simulink model "final_project_full_working"  (R2024b)
settings: Solver=ode1  StartTime=0.0  StopTime=5  RelTol=1e-4  AbsTol=1e-3
undefined symbols (not defined in the file): DiscIntNeverNeededParam, Ion, Lithium
libraries: spsSeriesRLCBranchLib x25, slpidlib x12, spsThreePhaseVIMeasurementLib x11, spsPower3phInstantaneousLib x9, spsIGBTDiodeLib x7, spsThreePhaseParallelRLCLoadLib x7, spsCurrentMeasurementLib x4, spsabctodq0Lib x3, spsVoltageMeasurementLib x3, spsGroundLib x3, spsVariableResistorLib x3, spsControlledVoltageSourceLib x3
(part 1 of 2)
settings Model: Creator=ALVEE  LastModifiedBy=ALVEE
settings SolverCC: SolverResetMethod=Robust

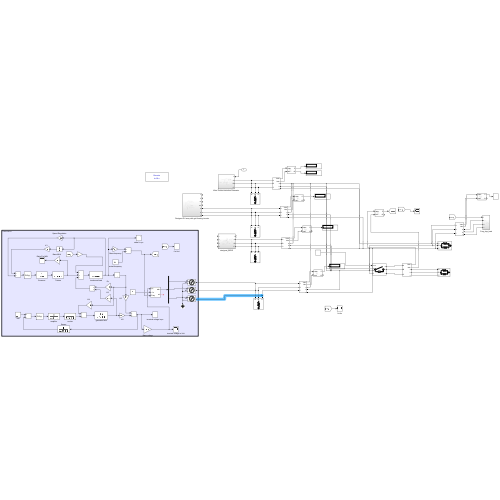
[thumbnail: Simulink's stored preview of the top-level diagram]
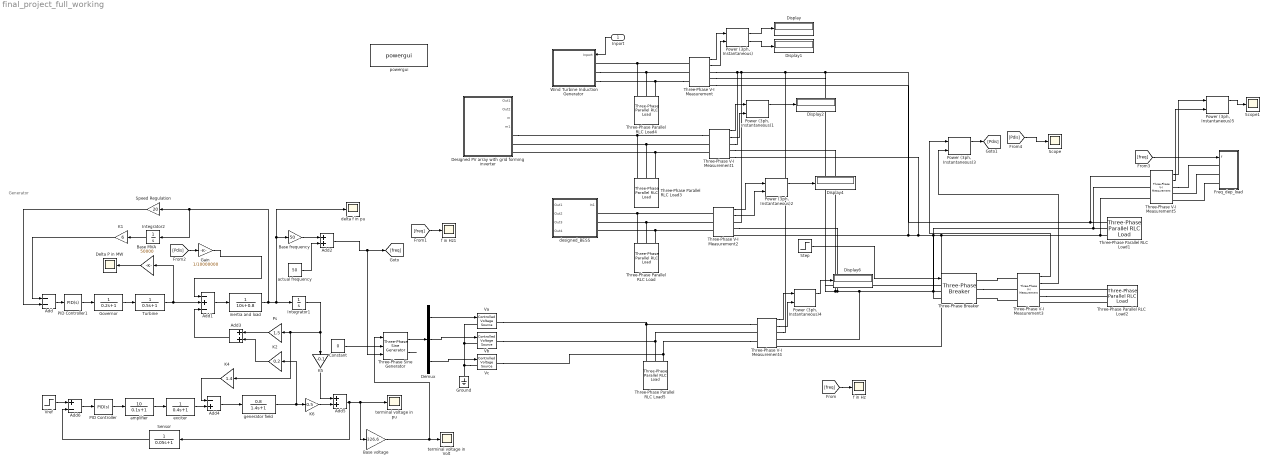
== system final_project_full_working ==
  note: Generator
  Inport : Inport
  Add : Sum  Inputs=--
  Add1 : Sum  Inputs=-+-
  Add2 : Sum
  Add3 : Sum
  Add4 : Sum  Inputs=-+
  Add5 : Sum
  Add6 : Sum  Inputs=+-
  Base MVA : Gain  Gain=50000
  Base frequency : Gain  Gain=50
  Base voltage : Gain  Gain=326.6
  Constant : Constant  Value=0
  Delta P in MW : Scope
  Demux : Demux  Outputs=3
  Designed PV array with grid forming inverter : Subsystem
  Display{,1..2,4,6} (5 alike) : Display
  Freq_dep_load : Subsystem
  Gain : Gain  Gain=1/10000000
  Governor : TransferFcn  Denominator=[0.2 1]
  Ground : spsGroundLib/Ground  LConnTagsString=a
  Integrator1 : Integrator
  Integrator2 : Integrator
  K1 : Gain  Gain=6
  K2 : Gain  Gain=0.2
  K4 : Gain  Gain=1.4
  K5 : Gain  Gain=-0.1
  K6 : Gain  Gain=0.5
  PID Controller : slpidlib/PID Controller  Controller=PID  Form=Parallel  TimeDomain=Continuous-time  UseExternalTs=off  SampleTime=-1  IntegratorMethod=Forward Euler  FilterMethod=Forward Euler  ControllerParametersSource=internal  P=1  I=0.25  UseKiTs=off  D=0.3  UseExternalDerivativeSource=off  N=100  UseFilter=on  TunerSelectOption=Transfer Function Based (PID Tuner App)  InitialConditionSource=internal  InitialConditionForIntegrator=0  InitialConditionForFilter=0  DifferentiatorICPrevScaledInput=0  ExternalReset=none  TrackingMode=off  Kt=1  LimitOutput=off  SatLimitsSource=internal  UpperSaturationLimit=inf  LowerSaturationLimit=-inf  LinearizeAsGain=on  AntiWindupMode=none  Kb=1  LimitIntegrator=off  UpperIntegratorSaturationLimit=inf  LowerIntegratorSaturationLimit=-inf  POutMin=[]  POutMax=[]  IOutMin=[]  IOutMax=[]  DOutMin=[]  DOutMax=[]  NOutMin=[]  NOutMax=[]  SumOutMin=[]  SumOutMax=[]  SaturationOutMin=[]  SaturationOutMax=[]  PParamMin=[]  PParamMax=[]  IParamMin=[]  IParamMax=[]  DParamMin=[]  DParamMax=[]  NParamMin=[]  NParamMax=[]  KbParamMin=[]  KbParamMax=[]  KtParamMin=[]  KtParamMax=[]  KbOutMin=[]  KbOutMax=[]  KtOutMin=[]  KtOutMax=[]  IntegratorOutMin=[]  IntegratorOutMax=[]  FilterOutMin=[]  FilterOutMax=[]  SumI1OutMin=[]  SumI1OutMax=[]  SumI2OutMin=[]  SumI2OutMax=[]  SumI3OutMin=[]  SumI3OutMax=[]  SumI4OutMin=[]  SumI4OutMax=[]  SumDOutMin=[]  SumDOutMax=[]  DifferentiatorOutMin=[]  DifferentiatorOutMax=[]  FilterDiffOutCoefMin=[]  FilterDiffOutCoefMax=[]  ReciprocalOutMin=[]  ReciprocalOutMax=[]  SumDenOutMin=[]  SumDenOutMax=[]  SumNumOutMin=[]  SumNumOutMax=[]  DivideOutMin=[]  DivideOutMax=[]  UdiffTsProdOutMin=[]  UdiffTsProdOutMax=[]  NTsProdOutMin=[]  NTsProdOutMax=[]  UintegralTsProdOutMin=[]  UintegralTsProdOutMax=[]  UngainTsProdOutMin=[]  UngainTsProdOutMax=[]  ClampingZeroOutDataTypeStr=Inherit: Inherit via back propagation  ClampingZeroOutMin=[]  ClampingZeroOutMax=[]  FilterDenConstantOutDataTypeStr=Inherit: Inherit via back propagation  FilterDenConstantOutMin=[]  FilterDenConstantOutMax=[]  PCopyOutDataTypeStr=Inherit: Inherit via back propagation  PCopyOutMin=[]  PCopyOutMax=[]  NCopyOutDataTypeStr=Inherit: Inherit via back propagation  NCopyOutMin=[]  NCopyOutMax=[]  IntegratorContinuousStateAttributes=''  IntegratorStateMustResolveToSignalObject=off  IntegratorRTWStateStorageClass=Auto  FilterContinuousStateAttributes=''  FilterStateMustResolveToSignalObject=off  FilterRTWStateStorageClass=Auto  ParallelPVariant=InternalParameters  IdealPVariant=Disabled  IVariant=InternalParameters  DVariant=InternalParameters  IntegratorVariant=Continuous  SatVariant=Disabled  AWVariant=Passthrough  PCopyVariant=Disabled  TRVariant=Disabled  FdbkBlocksVariant=Forward  IdealPFdbkVariant=Disabled  SatFdbkVariant=Disabled  DerivativeFilterVariant=ContFilter  NVariant=InternalParameters  NCopyVariant=Disabled  FilterICVariant=InternalICsFilter  IntegratorICVariant=InternalICs  ExternalResetVariant=Disabled  TRSumVariant=Passthrough  SumFdbkVariant=Disabled  SumVariant=Sum_PID  TsampFilterVariant=InternalTs  TsampNgainVariant=Passthrough  TsampIntegralVariant=Disabled_SignalSpec  ExternalSaturationOutDataTypeStr=Inherit: Same as second input  DerivativeSourceVariant=ErrorSignal  PreIntVariant=InternalPreInt
  PID Controller1 : slpidlib/PID Controller  Controller=PID  Form=Parallel  TimeDomain=Continuous-time  UseExternalTs=off  SampleTime=-1  IntegratorMethod=Forward Euler  FilterMethod=Forward Euler  ControllerParametersSource=internal  P=24.0972  I=15.6479  UseKiTs=off  D=10  UseExternalDerivativeSource=off  N=100  UseFilter=on  TunerSelectOption=Transfer Function Based (PID Tuner App)  InitialConditionSource=internal  InitialConditionForIntegrator=0  InitialConditionForFilter=0  DifferentiatorICPrevScaledInput=0  ExternalReset=none  TrackingMode=off  Kt=1  LimitOutput=off  SatLimitsSource=internal  UpperSaturationLimit=inf  LowerSaturationLimit=-inf  LinearizeAsGain=on  AntiWindupMode=none  Kb=1  LimitIntegrator=off  UpperIntegratorSaturationLimit=inf  LowerIntegratorSaturationLimit=-inf  POutMin=[]  POutMax=[]  IOutMin=[]  IOutMax=[]  DOutMin=[]  DOutMax=[]  NOutMin=[]  NOutMax=[]  SumOutMin=[]  SumOutMax=[]  SaturationOutMin=[]  SaturationOutMax=[]  PParamMin=[]  PParamMax=[]  IParamMin=[]  IParamMax=[]  DParamMin=[]  DParamMax=[]  NParamMin=[]  NParamMax=[]  KbParamMin=[]  KbParamMax=[]  KtParamMin=[]  KtParamMax=[]  KbOutMin=[]  KbOutMax=[]  KtOutMin=[]  KtOutMax=[]  IntegratorOutMin=[]  IntegratorOutMax=[]  FilterOutMin=[]  FilterOutMax=[]  SumI1OutMin=[]  SumI1OutMax=[]  SumI2OutMin=[]  SumI2OutMax=[]  SumI3OutMin=[]  SumI3OutMax=[]  SumI4OutMin=[]  SumI4OutMax=[]  SumDOutMin=[]  SumDOutMax=[]  DifferentiatorOutMin=[]  DifferentiatorOutMax=[]  FilterDiffOutCoefMin=[]  FilterDiffOutCoefMax=[]  ReciprocalOutMin=[]  ReciprocalOutMax=[]  SumDenOutMin=[]  SumDenOutMax=[]  SumNumOutMin=[]  SumNumOutMax=[]  DivideOutMin=[]  DivideOutMax=[]  UdiffTsProdOutMin=[]  UdiffTsProdOutMax=[]  NTsProdOutMin=[]  NTsProdOutMax=[]  UintegralTsProdOutMin=[]  UintegralTsProdOutMax=[]  UngainTsProdOutMin=[]  UngainTsProdOutMax=[]  ClampingZeroOutDataTypeStr=Inherit: Inherit via back propagation  ClampingZeroOutMin=[]  ClampingZeroOutMax=[]  FilterDenConstantOutDataTypeStr=Inherit: Inherit via back propagation  FilterDenConstantOutMin=[]  FilterDenConstantOutMax=[]  PCopyOutDataTypeStr=Inherit: Inherit via back propagation  PCopyOutMin=[]  PCopyOutMax=[]  NCopyOutDataTypeStr=Inherit: Inherit via back propagation  NCopyOutMin=[]  NCopyOutMax=[]  IntegratorContinuousStateAttributes=''  IntegratorStateMustResolveToSignalObject=off  IntegratorRTWStateStorageClass=Auto  FilterContinuousStateAttributes=''  FilterStateMustResolveToSignalObject=off  FilterRTWStateStorageClass=Auto  ParallelPVariant=InternalParameters  IdealPVariant=Disabled  IVariant=InternalParameters  DVariant=InternalParameters  IntegratorVariant=Continuous  SatVariant=Disabled  AWVariant=Passthrough  PCopyVariant=Disabled  TRVariant=Disabled  FdbkBlocksVariant=Forward  IdealPFdbkVariant=Disabled  SatFdbkVariant=Disabled  DerivativeFilterVariant=ContFilter  NVariant=InternalParameters  NCopyVariant=Disabled  FilterICVariant=InternalICsFilter  IntegratorICVariant=InternalICs  ExternalResetVariant=Disabled  TRSumVariant=Passthrough  SumFdbkVariant=Disabled  SumVariant=Sum_PID  TsampFilterVariant=InternalTs  TsampNgainVariant=Passthrough  TsampIntegralVariant=Disabled_SignalSpec  ExternalSaturationOutDataTypeStr=Inherit: Same as second input  DerivativeSourceVariant=ErrorSignal  PreIntVariant=InternalPreInt
  Power (3ph, Instantaneous){,1..5} (6 alike) : spsPower3phInstantaneousLib/Power (3ph, Instantaneous)
  Ps : Gain  Gain=1.5
  Scope : Scope
  Scope1 : Scope
  Sensor : TransferFcn  Denominator=[0.05 1]
  Speed Regulation : Gain  Gain=20
  Step : Step  Time=2.5  SampleTime=0
  Three-Phase Parallel RLC Load{,3..5} (4 alike) : spsThreePhaseParallelRLCLoadLib/Three-Phase Parallel RLC Load  LConnTagsString=A|B|C  Configuration=Y (grounded)  NominalVoltage=400  Vabc=[1e3 1e3 1e3]  Vabcp=[1e3 1e3 1e3]  NominalFrequency=50  UnbalancedPower=off  ActivePower=100  InductivePower=0  CapacitivePower=0  Pabc=[10e3 9e3 11e3]  QLabc=[100 90 110]  QCabc=[100 90 110]  Pabcp=[10e3 9e3 11e3]  QLabcp=[100 90 110]  QCabcp=[100 90 110]  Measurements=None  LoadType=constant Z
  Three-Phase Parallel RLC Load1 : spsThreePhaseParallelRLCLoadLib/Three-Phase Parallel RLC Load  LConnTagsString=A|B|C  Configuration=Y (grounded)  NominalVoltage=400  Vabc=[1e3 1e3 1e3]  Vabcp=[1e3 1e3 1e3]  NominalFrequency=50  UnbalancedPower=off  ActivePower=10e6  InductivePower=100  CapacitivePower=0  Pabc=[10e3 9e3 11e3]  QLabc=[100 90 110]  QCabc=[100 90 110]  Pabcp=[10e3 9e3 11e3]  QLabcp=[100 90 110]  QCabcp=[100 90 110]  Measurements=None  LoadType=constant PQ
  Three-Phase Parallel RLC Load2 : spsThreePhaseParallelRLCLoadLib/Three-Phase Parallel RLC Load  LConnTagsString=A|B|C  Configuration=Y (grounded)  NominalVoltage=400  Vabc=[1e3 1e3 1e3]  Vabcp=[1e3 1e3 1e3]  NominalFrequency=50  UnbalancedPower=off  ActivePower=2e6  InductivePower=100  CapacitivePower=0  Pabc=[10e3 9e3 11e3]  QLabc=[100 90 110]  QCabc=[100 90 110]  Pabcp=[10e3 9e3 11e3]  QLabcp=[100 90 110]  QCabcp=[100 90 110]  Measurements=None  LoadType=constant PQ
  Three-Phase Sine Generator : spsThreePhaseSineGeneratorLib/Three-Phase Sine Generator  Ts=0.0002
      settings: LibrarySourceBlock=|
      | sps_lib/Sources/Signal Generator Sources/Three-Phase
      | Sine Generator
  Three-Phase V-I Measurement{,1..5} (6 alike) : spsThreePhaseVIMeasurementLib/Three-Phase V-I Measurement  VoltageMeasurement=phase-to-ground  SetLabelV=off  LabelV=Vabc  Vpu=off  VpuLL=off  CurrentMeasurement=yes  SetLabelI=off  LabelI=Iabc  Ipu=off  Pbase=100e6  Vbase=500e3  OutputType=Complex  PhasorSimulation=off  PSBequivalent=0
  Three-Phase Breaker : spsThreePhaseBreakerLib/Three-Phase Breaker  InitialState=open  SwitchA=on  SwitchB=on  SwitchC=on  SwitchTimes="[1/60  5/60]"  External=on  BreakerResistance=0.01  SnubberResistance=1e6  SnubberCapacitance=inf  Measurements=None
  Turbine : TransferFcn  Denominator=[0.5 1]
  Va : spsControlledVoltageSourceLib/Controlled Voltage Source  Initialize=on  Source_Type=AC  Amplitude=0  Phase=0  Frequency=0  Measurements=None
  Vb : spsControlledVoltageSourceLib/Controlled Voltage Source  Initialize=on  Source_Type=AC  Amplitude=0  Phase=0  Frequency=0  Measurements=None
  Vc : spsControlledVoltageSourceLib/Controlled Voltage Source  Initialize=on  Source_Type=AC  Amplitude=0  Phase=0  Frequency=0  Measurements=None
  Vref : Step  Time=100  Before=1  SampleTime=0
  Wind Turbine Induction Generator : Subsystem
  actual frequency : Constant  Value=50
  amplifier : TransferFcn  Numerator=[10]  Denominator=[0.1 1]
  delta f in pu : Scope
  designed_BESS : Subsystem
  exciter : TransferFcn  Denominator=[0.4 1]
  f in Hz : Scope
  f in Hz1 : Scope
  generator field : TransferFcn  Numerator=[0.8]  Denominator=[1.4 1]
  inertia and load : TransferFcn  Denominator=[10 0.8]
  powergui : spspowerguiLib/powergui  Priority=1  SimulationMode=Discrete  SampleTime=1e-5  frequency=60  Iterations=50  frequencyindice=0  Pbase=100e6  ErrMax=1e-4  UnitsV=kV  UnitsW=MW  buscounter=0  FunctionMessages=off  echomessages=off  EnableUseOfTLC=off  CurrentSourceSwitches=off  DisableSnubberDevices=off  DisableRonSwitches=off  DisableVfSwitches=off  DisplayEquations=off  AutomaticDiscreteSolvers=off  SolverType=Tustin/Backward Euler (TBE)  Interpol=off  ExternalGateDelay=off  methode=off  Ts=100  x0status=blocks  SPID=on  SwTol=0  HookPort=off  NonlinearTolerance=1e-4  nMaxIteration=100  ContinueOnMaxIteration=off  RestoreLinks=warning  ResistiveCurrentMeasurement=off  Frange=[0:2:500]  Ylog=off  Xlog=on  ShowGrid=off  save=off  variable=ZData  structure=0  ZoomFFT=off  StartTime=0.0  cycles=1  DisplayStyle=1  fundamental=60  FreqAxis=off  MaxFrequency=1000  frequencyindicesteady=1  RmsSteady=1  display=off
  terminal voltage in Volt : Scope
  terminal voltage in pu : Scope
  wires:
  Three-Phase Sine Generator/2 -> ?
  Add3/1 -> Add1/3
  actual frequency/1 -> Add2/2
  inertia and load/1 -> Base frequency/1, delta f in pu/1, Integrator1/1, Speed Regulation/1, Integrator2/1
  K6/1 -> Add5/2
  Three-Phase V-I Measurement3/1 -> "Power (3ph, Instantaneous)3"/1
  PID Controller/1 -> amplifier/1
  Demux/3 -> Vc/1
  K2/1 -> Add3/2
  Base MVA/1 -> Delta P in MW/1
  Governor/1 -> Turbine/1
  Three-Phase V-I Measurement2/2 -> "Power (3ph, Instantaneous)2"/2
  Demux/2 -> Vb/1
  Sensor/1 -> Add6/2
  "Power (3ph, Instantaneous)"/2 -> Display1/1
  [freq] -> f in Hz1/1
  [Pdis] -> Gain/1
  Add4/1 -> generator field/1
  Integrator2/1 -> K1/1
  Turbine/1 -> Add1/2, Base MVA/1
  "Power (3ph, Instantaneous)"/1 -> Display/1
  Three-Phase V-I Measurement1/2 -> "Power (3ph, Instantaneous)1"/2
  Speed Regulation/1 -> Add/2
  Inport/1 -> Wind Turbine Induction Generator/1(Inport)
  Three-Phase Sine Generator/1 -> Demux/1
  "Power (3ph, Instantaneous)4"/1 -> Display6/1
  [Pdis] -> Scope/1
  "Power (3ph, Instantaneous)2"/1 -> Display4/1
  K4/1 -> Add4/1
  Integrator1/1 -> K5/1, K4/1, Ps/1
  "Power (3ph, Instantaneous)1"/1 -> Display2/1
  generator field/1 -> K2/1, K6/1
  "Power (3ph, Instantaneous)3"/1 -> [Pdis]
  Three-Phase V-I Measurement1/1 -> "Power (3ph, Instantaneous)1"/1
  Add2/1 -> Three-Phase Sine Generator/3, [freq]
  Constant/1 -> Three-Phase Sine Generator/2
  Three-Phase V-I Measurement/1 -> "Power (3ph, Instantaneous)"/1
  Three-Phase V-I Measurement2/1 -> "Power (3ph, Instantaneous)2"/1
  exciter/1 -> Add4/2
  Three-Phase V-I Measurement4/1 -> "Power (3ph, Instantaneous)4"/1
  Base frequency/1 -> Add2/1
  Ps/1 -> Add3/1
  [freq] -> Freq_dep_load/1(f)
  Three-Phase V-I Measurement4/2 -> "Power (3ph, Instantaneous)4"/2
  Base voltage/1 -> Three-Phase Sine Generator/1, terminal voltage in Volt/1
  Gain/1 -> Add1/1
  Vref/1 -> Add6/1
  [freq] -> f in Hz/1
  Add1/1 -> inertia and load/1
  Demux/1 -> Va/1
  K1/1 -> Add/1
  Add6/1 -> PID Controller/1
  Three-Phase V-I Measurement3/2 -> "Power (3ph, Instantaneous)3"/2
  Add5/1 -> Base voltage/1, terminal voltage in pu/1, Sensor/1
  Three-Phase V-I Measurement5/1 -> "Power (3ph, Instantaneous)5"/1
  "Power (3ph, Instantaneous)5"/1 -> Scope1/1
  Three-Phase V-I Measurement/2 -> "Power (3ph, Instantaneous)"/2
  Three-Phase V-I Measurement5/2 -> "Power (3ph, Instantaneous)5"/2
  Step/1 -> Three-Phase Breaker/1
  amplifier/1 -> exciter/1
  K5/1 -> Add5/1
  Add/1 -> PID Controller1/1
  PID Controller1/1 -> Governor/1
  connections:
  Three-Phase Parallel RLC Load3/LConn3 -- Three-Phase V-I Measurement1/LConn3 -- Designed PV array with grid forming inverter/RConn3
  Three-Phase V-I Measurement1/RConn3 -- Three-Phase Breaker/LConn3 -- Three-Phase V-I Measurement5/LConn3 -- Three-Phase Parallel RLC Load1/LConn3 -- Three-Phase V-I Measurement4/RConn3 -- Three-Phase V-I Measurement/RConn3 -- Three-Phase V-I Measurement2/RConn3
  Three-Phase V-I Measurement/LConn3 -- Wind Turbine Induction Generator/LConn3 -- Three-Phase Parallel RLC Load4/LConn3
  Three-Phase V-I Measurement2/RConn1 -- Three-Phase V-I Measurement5/LConn1 -- Three-Phase Parallel RLC Load1/LConn1 -- Three-Phase Breaker/LConn1 -- Three-Phase V-I Measurement4/RConn1 -- Three-Phase V-I Measurement/RConn1 -- Three-Phase V-I Measurement1/RConn1
  Three-Phase V-I Measurement4/LConn3 -- Three-Phase Parallel RLC Load5/LConn3 -- Vc/RConn1
  Vc/LConn1 -- Va/LConn1 -- Vb/LConn1 -- Ground/LConn1
  Three-Phase V-I Measurement2/RConn2 -- Three-Phase V-I Measurement5/LConn2 -- Three-Phase Parallel RLC Load1/LConn2 -- Three-Phase Breaker/LConn2 -- Three-Phase V-I Measurement4/RConn2 -- Three-Phase V-I Measurement/RConn2 -- Three-Phase V-I Measurement1/RConn2
  Three-Phase V-I Measurement4/LConn1 -- Three-Phase Parallel RLC Load5/LConn1 -- Va/RConn1
  designed_BESS/LConn1 -- Three-Phase V-I Measurement2/LConn1 -- Three-Phase Parallel RLC Load/LConn1
  Three-Phase Parallel RLC Load/LConn2 -- Three-Phase V-I Measurement2/LConn2 -- designed_BESS/LConn2
  Three-Phase V-I Measurement1/LConn1 -- Designed PV array with grid forming inverter/RConn1 -- Three-Phase Parallel RLC Load3/LConn1
  Three-Phase Parallel RLC Load/LConn3 -- Three-Phase V-I Measurement2/LConn3 -- designed_BESS/LConn3
  Three-Phase Parallel RLC Load4/LConn2 -- Wind Turbine Induction Generator/LConn2 -- Three-Phase V-I Measurement/LConn2
  Wind Turbine Induction Generator/LConn1 -- Three-Phase V-I Measurement/LConn1 -- Three-Phase Parallel RLC Load4/LConn1
  Three-Phase Parallel RLC Load3/LConn2 -- Three-Phase V-I Measurement1/LConn2 -- Designed PV array with grid forming inverter/RConn2
  Vb/RConn1 -- Three-Phase V-I Measurement4/LConn2 -- Three-Phase Parallel RLC Load5/LConn2
  Three-Phase Breaker/RConn2 -- Three-Phase V-I Measurement3/LConn2
  Freq_dep_load/LConn3 -- Three-Phase V-I Measurement5/RConn3
  Three-Phase Parallel RLC Load2/LConn3 -- Three-Phase V-I Measurement3/RConn3
  Three-Phase V-I Measurement3/LConn1 -- Three-Phase Breaker/RConn1
  Three-Phase V-I Measurement5/RConn1 -- Freq_dep_load/LConn1
  Three-Phase Parallel RLC Load2/LConn1 -- Three-Phase V-I Measurement3/RConn1
  Three-Phase V-I Measurement3/LConn3 -- Three-Phase Breaker/RConn3
  Three-Phase V-I Measurement3/RConn2 -- Three-Phase Parallel RLC Load2/LConn2
  Freq_dep_load/LConn2 -- Three-Phase V-I Measurement5/RConn2

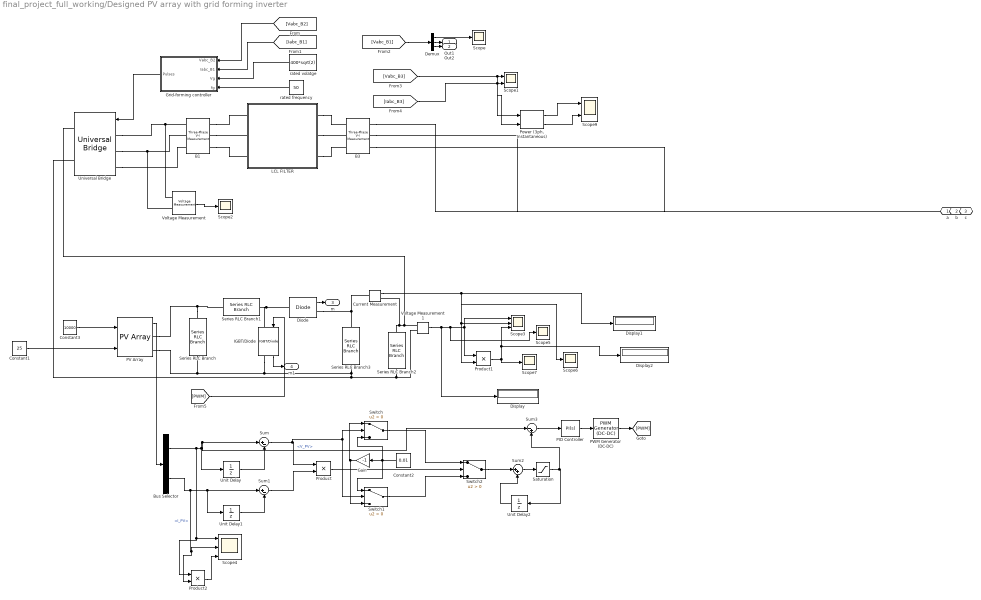
== system final_project_full_working/Designed PV array with grid forming inverter ==
  B1 : spsThreePhaseVIMeasurementLib/Three-Phase V-I Measurement  VoltageMeasurement=phase-to-ground  SetLabelV=on  LabelV=Vabc_B1  Vpu=off  VpuLL=off  CurrentMeasurement=yes  SetLabelI=on  LabelI=Iabc_B1  Ipu=off  Pbase=100e6  Vbase=500e3  OutputType=Complex  PhasorSimulation=off  PSBequivalent=0
  B3 : spsThreePhaseVIMeasurementLib/Three-Phase V-I Measurement  VoltageMeasurement=phase-to-ground  SetLabelV=on  LabelV=Vabc_B3  Vpu=off  VpuLL=off  CurrentMeasurement=yes  SetLabelI=on  LabelI=Iabc_B3  Ipu=off  Pbase=100e6  Vbase=500e3  OutputType=Complex  PhasorSimulation=off  PSBequivalent=0
  Bus Selector : BusSelector  OutputSignals=V_PV,I_PV
  Constant1 : Constant  Value=25
  Constant2 : Constant  Value=0.01
  Constant3 : Constant  Value=10000
  Current Measurement : spsCurrentMeasurementLib/Current Measurement  PhasorSimulation=off  OutputType=Complex  PSBequivalent=0
  Demux : Demux  Outputs=3
  Diode : spsDiodeLib/Diode  Ron=0.01  Lon=0  Vf=0.8  IC=0  UseSnubber=0  Rs=500  Cs=250e-9  Measurements=on
  Display : Display
  Display1 : Display
  Display2 : Display
  Gain : Gain  Gain=-1
  Grid-forming controller : Subsystem
  IGBT/Diode : spsIGBTDiodeLib/IGBT//Diode  Ron=1e-3  Rs=1e5  Cs=inf  Measurements=on
  LCL FILTER : Subsystem
  PID Controller : slpidlib/PID Controller  Controller=PI  Form=Parallel  TimeDomain=Continuous-time  UseExternalTs=off  SampleTime=-1  IntegratorMethod=Forward Euler  FilterMethod=Forward Euler  ControllerParametersSource=internal  P=1  I=1  UseKiTs=off  D=0  UseExternalDerivativeSource=off  N=100  UseFilter=on  TunerSelectOption=Transfer Function Based (PID Tuner App)  InitialConditionSource=internal  InitialConditionForIntegrator=0  InitialConditionForFilter=0  DifferentiatorICPrevScaledInput=0  ExternalReset=none  TrackingMode=off  Kt=1  LimitOutput=off  SatLimitsSource=internal  UpperSaturationLimit=inf  LowerSaturationLimit=-inf  LinearizeAsGain=on  AntiWindupMode=none  Kb=1  LimitIntegrator=off  UpperIntegratorSaturationLimit=inf  LowerIntegratorSaturationLimit=-inf  POutMin=[]  POutMax=[]  IOutMin=[]  IOutMax=[]  DOutMin=[]  DOutMax=[]  NOutMin=[]  NOutMax=[]  SumOutMin=[]  SumOutMax=[]  SaturationOutMin=[]  SaturationOutMax=[]  PParamMin=[]  PParamMax=[]  IParamMin=[]  IParamMax=[]  DParamMin=[]  DParamMax=[]  NParamMin=[]  NParamMax=[]  KbParamMin=[]  KbParamMax=[]  KtParamMin=[]  KtParamMax=[]  KbOutMin=[]  KbOutMax=[]  KtOutMin=[]  KtOutMax=[]  IntegratorOutMin=[]  IntegratorOutMax=[]  FilterOutMin=[]  FilterOutMax=[]  SumI1OutMin=[]  SumI1OutMax=[]  SumI2OutMin=[]  SumI2OutMax=[]  SumI3OutMin=[]  SumI3OutMax=[]  SumI4OutMin=[]  SumI4OutMax=[]  SumDOutMin=[]  SumDOutMax=[]  DifferentiatorOutMin=[]  DifferentiatorOutMax=[]  FilterDiffOutCoefMin=[]  FilterDiffOutCoefMax=[]  ReciprocalOutMin=[]  ReciprocalOutMax=[]  SumDenOutMin=[]  SumDenOutMax=[]  SumNumOutMin=[]  SumNumOutMax=[]  DivideOutMin=[]  DivideOutMax=[]  UdiffTsProdOutMin=[]  UdiffTsProdOutMax=[]  NTsProdOutMin=[]  NTsProdOutMax=[]  UintegralTsProdOutMin=[]  UintegralTsProdOutMax=[]  UngainTsProdOutMin=[]  UngainTsProdOutMax=[]  ClampingZeroOutDataTypeStr=Inherit: Inherit via back propagation  ClampingZeroOutMin=[]  ClampingZeroOutMax=[]  FilterDenConstantOutDataTypeStr=Inherit: Inherit via back propagation  FilterDenConstantOutMin=[]  FilterDenConstantOutMax=[]  PCopyOutDataTypeStr=Inherit: Inherit via back propagation  PCopyOutMin=[]  PCopyOutMax=[]  NCopyOutDataTypeStr=Inherit: Inherit via back propagation  NCopyOutMin=[]  NCopyOutMax=[]  IntegratorContinuousStateAttributes=''  IntegratorStateMustResolveToSignalObject=off  IntegratorRTWStateStorageClass=Auto  FilterContinuousStateAttributes=''  FilterStateMustResolveToSignalObject=off  FilterRTWStateStorageClass=Auto  ParallelPVariant=InternalParameters  IdealPVariant=Disabled  IVariant=InternalParameters  DVariant=Disabled  IntegratorVariant=Continuous  SatVariant=Disabled  AWVariant=Passthrough  PCopyVariant=Disabled  TRVariant=Disabled  FdbkBlocksVariant=Forward  IdealPFdbkVariant=Disabled  SatFdbkVariant=Disabled  DerivativeFilterVariant=Disabled  NVariant=Disabled  NCopyVariant=Disabled_SignalSpec  FilterICVariant=Disabled  IntegratorICVariant=InternalICs  ExternalResetVariant=Disabled  TRSumVariant=Passthrough  SumFdbkVariant=Disabled  SumVariant=Sum_PI  TsampFilterVariant=InternalTs  TsampNgainVariant=Passthrough  TsampIntegralVariant=Disabled_SignalSpec  ExternalSaturationOutDataTypeStr=Inherit: Same as second input  DerivativeSourceVariant=Disabled  PreIntVariant=InternalPreInt
  PV Array : spsPVArrayLib/PV Array  Npar=1000  Nser=100  PlotType=array @ 25 deg.C & specified irradiances  S_vec="[ 1000  500  100 ]"  Temp_C_vec="[ 45 25  ]"  ModuleName=SunPower SPR-445J-WHT-D  PlotWhenSelected=off  Pm=444.86  Ncell=128  Voc=90.5  Isc=6.21  Vm=76.7  Im=5.8  beta_Voc_pc=-0.291  alpha_Isc_pc=0.013301  beta_Voc=-0.26336  alpha_Isc=0.000826  IL=6.2167  I0=1.3548e-11  nI=1.026  Rsh=508.2885  Rs=0.54863  RobustModel=off  RobustCellTemperature=313.3991  BAL=on  Tc=1e-6  Tfilter=5e-5
  PWM Generator (DC-DC) : spsPWMGeneratorDCDCLib/PWM Generator (DC-DC)  Fsw=10000  Ts=0
  "Power (3ph, Instantaneous)" : spsPower3phInstantaneousLib/Power (3ph, Instantaneous)
  Product : Product
  Product1 : Product
  Product2 : Product
  Saturation : Saturate  UpperLimit=400  LowerLimit=350
  Scope{,2,5..7} (5 alike) : Scope
  Scope1 : Scope  NumInputPorts=2
  Scope3 : Scope  NumInputPorts=3
  Scope4 : Scope  NumInputPorts=3
  Scope9 : Scope  NumInputPorts=2
  Series RLC Branch : spsSeriesRLCBranchLib/Series RLC Branch  LConnTagsString=__new0  RConnTagsString=__new0  BranchType=C  Resistance=1  Inductance=1e-3  SetiL0=off  InitialCurrent=0  Capacitance=1.5625e-3  Setx0=off  InitialVoltage=0  Measurements=None
  Series RLC Branch1 : spsSeriesRLCBranchLib/Series RLC Branch  LConnTagsString=__new0  RConnTagsString=__new0  BranchType=L  Resistance=1  Inductance=0.1024  SetiL0=off  InitialCurrent=0  Capacitance=1e-6  Setx0=off  InitialVoltage=0  Measurements=None
  Series RLC Branch2 : spsSeriesRLCBranchLib/Series RLC Branch  LConnTagsString=__new0  RConnTagsString=__new0  BranchType=R  Resistance=0.15994  Inductance=1e-3  SetiL0=off  InitialCurrent=0  Capacitance=1e-6  Setx0=off  InitialVoltage=0  Measurements=None
  Series RLC Branch3 : spsSeriesRLCBranchLib/Series RLC Branch  LConnTagsString=__new0  RConnTagsString=__new0  BranchType=C  Resistance=1  Inductance=1e-3  SetiL0=off  InitialCurrent=0  Capacitance=0.015625  Setx0=off  InitialVoltage=0  Measurements=None
  Sum : Sum  Inputs=|+-
  Sum1 : Sum  Inputs=|+-
  Sum2 : Sum  Inputs=|++
  Sum3 : Sum  Inputs=|-+
  Switch : Switch  Criteria=u2 > Threshold  SaturateOnIntegerOverflow=off  InputSameDT=off
  Switch1 : Switch  Criteria=u2 > Threshold  SaturateOnIntegerOverflow=off  InputSameDT=off
  Switch2 : Switch  Criteria=u2 > Threshold  SaturateOnIntegerOverflow=off  InputSameDT=off
  Unit Delay : UnitDelay  SampleTime=-1  HasFrameUpgradeWarning=on
  Unit Delay1 : UnitDelay  SampleTime=-1  HasFrameUpgradeWarning=on
  Unit Delay2 : UnitDelay  SampleTime=-1  HasFrameUpgradeWarning=on
  Universal Bridge : spsUniversalBridgeLib/Universal Bridge  Arms=3  SnubberResistance=1e5  SnubberCapacitance=inf  Device=IGBT / Diodes  Ron=1e-3  Lon=0  ForwardVoltages="[  0  0  ]"  ForwardVoltage=0  GTOparameters=[ 10e-6 , 20e-6 ]  IGBTparameters=[ 1e-6 , 2e-6 ]  Measurements=None  Measurements_2=None  converterType=Rectifier
  Voltage Measurement : spsVoltageMeasurementLib/Voltage Measurement  PhasorSimulation=off  OutputType=Complex  PSBequivalent=0
  Voltage Measurement1 : spsVoltageMeasurementLib/Voltage Measurement  PhasorSimulation=off  OutputType=Complex  PSBequivalent=0
  rated frequency : Constant  Value=50  SampleTime=10e-6
  rated volatge : Constant  Value=400*sqrt(2)  SampleTime=10e-6
  a : PMIOPort  Side=Right
  b : PMIOPort  Port=2  Side=Right
  c : PMIOPort  Port=3  Side=Right
  Out1 : Outport
  Out2 : Outport  Port=2
  m : Outport  Port=3
  m1 : Outport  Port=4
  wires:
  Bus Selector/1 -> Product2/1, Scope4/1, Unit Delay/1, Sum3/1, Sum/1  "<V_PV>"
  Current Measurement/1 -> Display1/1, Product1/2, Scope3/2, Scope6/1
  Product/1 -> Switch2/2
  Demux/1 -> Scope/1
  Product1/1 -> Display2/1, Scope3/3, Scope7/1
  Constant2/1 -> Switch1/1, Switch/3, Gain/1
  Sum/1 -> Switch1/2, Switch/2, Product/1
  [Vabc_B2] -> Grid-forming controller/1(Vabc_B2)
  Sum3/1 -> PID Controller/1
  rated volatge/1 -> Grid-forming controller/3(Vg)
  Voltage Measurement1/1 -> Display/1, Scope5/1, Scope3/1, Product1/1
  [Iabc_B3] -> "Power (3ph, Instantaneous)"/2, Scope1/2
  "Power (3ph, Instantaneous)"/2 -> Scope9/2
  Bus Selector/2 -> Product2/2, Scope4/2, Unit Delay1/1, Sum1/1  "<I_PV>"
  Unit Delay/1 -> Sum/2
  PID Controller/1 -> PWM Generator (DC-DC)/1
  [Iabc_B1] -> Grid-forming controller/2(Iabc_B1)
  Gain/1 -> Switch1/3, Switch/1
  [PWM] -> IGBT/Diode/1
  Unit Delay2/1 -> Sum2/2
  Grid-forming controller/1(Pulses) -> Universal Bridge/1
  PV Array/1 -> Bus Selector/1
  Switch2/1 -> Sum2/1
  Saturation/1 -> Sum3/2, Unit Delay2/1
  Constant3/1 -> PV Array/1
  [Vabc_B3] -> "Power (3ph, Instantaneous)"/1, Scope1/1
  PWM Generator (DC-DC)/1 -> [PWM]
  "Power (3ph, Instantaneous)"/1 -> Scope9/1
  Diode/1 -> m/1
  Unit Delay1/1 -> Sum1/2
  Constant1/1 -> PV Array/2
  [Vabc_B1] -> Demux/1
  Demux/2 -> Out1/1
  Switch/1 -> Switch2/1
  Product2/1 -> Scope4/3
  Demux/3 -> Out2/1
  rated frequency/1 -> Grid-forming controller/4(fg)
  Switch1/1 -> Switch2/3
  IGBT/Diode/1 -> m1/1
  Voltage Measurement/1 -> Scope2/1
  Sum1/1 -> Product/2
  Sum2/1 -> Saturation/1
  connections:
  Series RLC Branch2/RConn1 -- Universal Bridge/RConn2 -- Series RLC Branch3/RConn1 -- IGBT/Diode/RConn1 -- PV Array/RConn2 -- Series RLC Branch/RConn1 -- Voltage Measurement1/LConn2
  Universal Bridge/LConn2 -- Voltage Measurement/LConn2 -- B1/LConn2
  Diode/RConn1 -- Current Measurement/LConn1 -- Series RLC Branch3/LConn1
  Series RLC Branch/LConn1 -- PV Array/RConn1 -- Series RLC Branch1/LConn1
  Universal Bridge/LConn3 -- B1/LConn3
  B1/RConn3 -- LCL FILTER/LConn3
  B3/RConn2 -- b/RConn1
  Diode/LConn1 -- IGBT/Diode/LConn1 -- Series RLC Branch1/RConn1
  B3/RConn1 -- a/RConn1
  Universal Bridge/LConn1 -- Voltage Measurement/LConn1 -- B1/LConn1
  LCL FILTER/RConn1 -- B3/LConn1
  LCL FILTER/RConn2 -- B3/LConn2
  B1/RConn1 -- LCL FILTER/LConn1
  B1/RConn2 -- LCL FILTER/LConn2
  LCL FILTER/RConn3 -- B3/LConn3
  Current Measurement/RConn1 -- Universal Bridge/RConn1 -- Voltage Measurement1/LConn1 -- Series RLC Branch2/LConn1
  B3/RConn3 -- c/RConn1

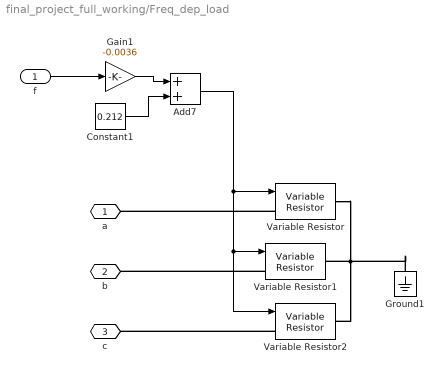
== system final_project_full_working/Freq_dep_load ==
  f : Inport
  Add7 : Sum
  Constant1 : Constant  Value=0.212
  Gain1 : Gain  Gain=-0.0036
  Ground1 : spsGroundLib/Ground  LConnTagsString=a
  Variable Resistor : spsVariableResistorLib/Variable Resistor  Rabsmin=1e-3
  Variable Resistor1 : spsVariableResistorLib/Variable Resistor  Rabsmin=1e-3
  Variable Resistor2 : spsVariableResistorLib/Variable Resistor  Rabsmin=1e-3
  a : PMIOPort  Side=Left
  " b" : PMIOPort  Port=2  Side=Left
  " c" : PMIOPort  Port=3  Side=Left
  wires:
  f/1 -> Gain1/1
  Constant1/1 -> Add7/2
  Add7/1 -> Variable Resistor2/1, Variable Resistor1/1, Variable Resistor/1
  Gain1/1 -> Add7/1
  connections:
  Variable Resistor/RConn1 -- Variable Resistor2/RConn1 -- Ground1/LConn1 -- Variable Resistor1/RConn1
  Variable Resistor2/LConn1 -- " c"/RConn1
  Variable Resistor/LConn1 -- a/RConn1
  Variable Resistor1/LConn1 -- " b"/RConn1

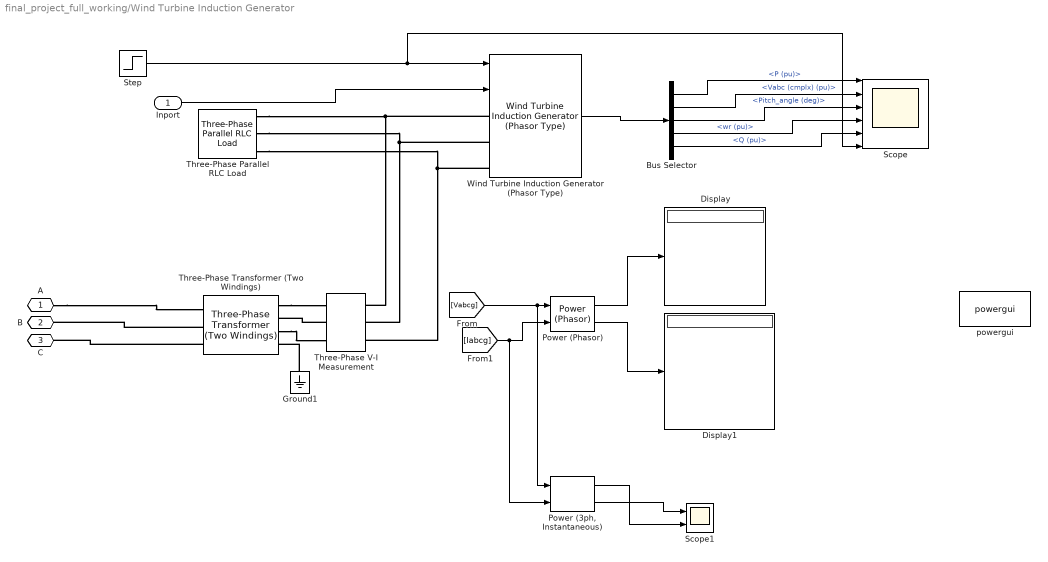
== system final_project_full_working/Wind Turbine Induction Generator ==
  Inport : Inport
  Bus Selector : BusSelector  OutputSignals=P (pu),Vabc (cmplx) (pu),Pitch_angle (deg),wr (pu),Q (pu)
  Display : Display
  Display1 : Display
  Ground1 : spsGroundLib/Ground  LConnTagsString=a
  "Power (3ph, Instantaneous)" : spsPower3phInstantaneousLib/Power (3ph, Instantaneous)
  Power (Phasor) : spsPowerPhasorLib/Power (Phasor)
  Scope : Scope  NumInputPorts=6
  Scope1 : Scope  NumInputPorts=2
  Step : Step  Time=2.5  Before=12  After=12.5  SampleTime=0
  Three-Phase Parallel RLC Load : spsThreePhaseParallelRLCLoadLib/Three-Phase Parallel RLC Load  LConnTagsString=A|B|C  Configuration=Y (grounded)  NominalVoltage=400  Vabc=[1e3 1e3 1e3]  Vabcp=[1e3 1e3 1e3]  NominalFrequency=50  UnbalancedPower=off  ActivePower=0  InductivePower=0  CapacitivePower=5000  Pabc=[10e3 9e3 11e3]  QLabc=[100 90 110]  QCabc=[100 90 110]  Pabcp=[10e3 9e3 11e3]  QLabcp=[100 90 110]  QCabcp=[100 90 110]  Measurements=None  LoadType=constant Z
  Three-Phase Transformer (Two Windings) : spsThreePhaseTransformerTwoWindingsLib/Three-Phase Transformer (Two Windings)  Winding1Connection=Yg  Winding2Connection=Yn  CoreType=Three single-phase transformers  SetSaturation=off  Hysteresis=off  DataFile='hysteresis'  SetInitialFlux=off  Measurements=None  UNITS=pu  NominalPower=[ 15e3 , 50 ]  Winding1=[ 400 , 0.002 , 0.08 ]  Winding2=[ 400 , 0.002 , 0.08 ]  Rm=500  Lm=inf  L0=0.5  Saturation=[ 0,0 ; 0.0024,1.2 ; 1.0,1.52 ]  InitialFluxes=[ 0.8 , -0.8 , 0.7 ]  BreakLoop=off  DiscreteSolver=Trapezoidal iterative  DataType=off  TransfoNumber=1
  Three-Phase V-I Measurement : spsThreePhaseVIMeasurementLib/Three-Phase V-I Measurement  VoltageMeasurement=phase-to-ground  SetLabelV=on  LabelV=Vabcg  Vpu=off  VpuLL=off  CurrentMeasurement=yes  SetLabelI=on  LabelI=Iabcg  Ipu=off  Pbase=100e6  Vbase=500e3  OutputType=Complex  PhasorSimulation=off  PSBequivalent=0
  Wind Turbine Induction Generator (Phasor Type) : spsWindTurbineInductionGeneratorPhasorTypeLib/Wind Turbine Induction Generator (Phasor Type)  ExternalTm=off  nom=[10e3, 400, 50]  sta=[ 0.004843, 0.1248]  rot=[ 0.004377, 0.1791]  Lm=6.77  mec=[5.04, 0.01, 3]  init="[ -0.01,0,   0,0,0,   0,0,0 ]"  pitch_angle=0  Pmec=1e4  wind_base=12  speed_nom=1  P_wind_base=1  K_pitch_gain=[5 25]  pitch_max=45  pitch_rate=2
  powergui : spspowerguiLib/powergui  Priority=1  SimulationMode=Discrete  SampleTime=1e-5  frequency=50  Iterations=50  frequencyindice=50  Pbase=100e6  ErrMax=1e-4  UnitsV=kV  UnitsW=MW  buscounter=0  FunctionMessages=off  echomessages=off  EnableUseOfTLC=off  CurrentSourceSwitches=off  DisableSnubberDevices=off  DisableRonSwitches=off  DisableVfSwitches=off  DisplayEquations=off  AutomaticDiscreteSolvers=off  SolverType=Tustin/Backward Euler (TBE)  Interpol=off  ExternalGateDelay=off  methode=off  Ts=100  x0status=blocks  SPID=on  SwTol=0  HookPort=off  NonlinearTolerance=1e-4  nMaxIteration=100  ContinueOnMaxIteration=off  RestoreLinks=warning  ResistiveCurrentMeasurement=off  Frange=[0:2:500]  Ylog=off  Xlog=on  ShowGrid=off  save=off  variable=ZData  structure=0  ZoomFFT=off  StartTime=0.0  cycles=1  DisplayStyle=1  fundamental=60  FreqAxis=off  MaxFrequency=1000  frequencyindicesteady=1  RmsSteady=1  display=off
  A : PMIOPort  Side=Left
  B : PMIOPort  Port=2  Side=Left
  C : PMIOPort  Port=3  Side=Left
  wires:
  Bus Selector/5 -> Scope/5  "<Q (pu)>"
  Bus Selector/1 -> Scope/1  "<P (pu)>"
  Wind Turbine Induction Generator (Phasor Type)/1 -> Bus Selector/1
  Power (Phasor)/2 -> Display1/1
  [Iabcg] -> "Power (3ph, Instantaneous)"/2, Power (Phasor)/2
  [Vabcg] -> "Power (3ph, Instantaneous)"/1, Power (Phasor)/1
  Bus Selector/3 -> Scope/3  "<Pitch_angle (deg)>"
  Step/1 -> Scope/6, Wind Turbine Induction Generator (Phasor Type)/1
  Power (Phasor)/1 -> Display/1
  Inport/1 -> Wind Turbine Induction Generator (Phasor Type)/2
  Bus Selector/2 -> Scope/2  "<Vabc (cmplx) (pu)>"
  Bus Selector/4 -> Scope/4  "<wr (pu)>"
  "Power (3ph, Instantaneous)"/1 -> Scope1/2
  "Power (3ph, Instantaneous)"/2 -> Scope1/1
  connections:
  Three-Phase Transformer (Two Windings)/RConn1 -- Three-Phase V-I Measurement/LConn1
  Ground1/LConn1 -- Three-Phase Transformer (Two Windings)/RConn4
  Wind Turbine Induction Generator (Phasor Type)/LConn3 -- Three-Phase Parallel RLC Load/LConn3 -- Three-Phase V-I Measurement/RConn3
  A/RConn1 -- Three-Phase Transformer (Two Windings)/LConn1
  Wind Turbine Induction Generator (Phasor Type)/LConn2 -- Three-Phase Parallel RLC Load/LConn2 -- Three-Phase V-I Measurement/RConn2
  Three-Phase Transformer (Two Windings)/RConn3 -- Three-Phase V-I Measurement/LConn3
  Wind Turbine Induction Generator (Phasor Type)/LConn1 -- Three-Phase Parallel RLC Load/LConn1 -- Three-Phase V-I Measurement/RConn1
  Three-Phase V-I Measurement/LConn2 -- Three-Phase Transformer (Two Windings)/RConn2
  Three-Phase Transformer (Two Windings)/LConn2 -- B/RConn1
  Three-Phase Transformer (Two Windings)/LConn3 -- C/RConn1
